simulink model "pilote_proportionnel_archive"  (R2018b)
settings: Solver=VariableStepAuto  StartTime=0.0  StopTime=10  MaxStep=0.01  RelTol=1e-3
undefined symbols (not defined in the file): alpha, beta, k, to
settings Model: Creator=12210406  LastModifiedBy=12210406

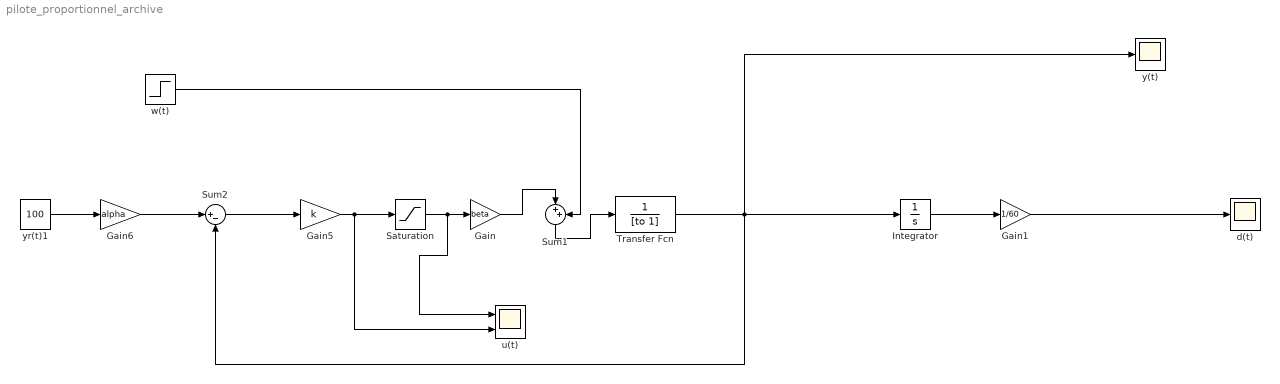
== system pilote_proportionnel_archive ==
  Gain : Gain  Gain=beta
  Gain1 : Gain  Gain=1/60
  Gain5 : Gain  Gain=k
  Gain6 : Gain  Gain=alpha
  Integrator : Integrator  LimitOutput=on  UpperSaturationLimit=t  LowerSaturationLimit=0
  Saturation : Saturate  UpperLimit=100  LowerLimit=-50
  Sum1 : Sum  Inputs=|++
  Sum2 : Sum  Inputs=|+-
  Transfer Fcn : TransferFcn  Denominator=[to 1]
  d(t) : Scope
  u(t) : Scope  NumInputPorts=2
  "w(t) " : Step  After=-10  SampleTime=0
  y(t) : Scope
  yr(t)1 : Constant  Value=100
  wires:
  Transfer Fcn/1 -> y(t)/1, Integrator/1, Sum2/2
  Integrator/1 -> Gain1/1
  Gain1/1 -> d(t)/1
  Saturation/1 -> u(t)/1, Gain/1
  Gain6/1 -> Sum2/1
  yr(t)1/1 -> Gain6/1
  Sum2/1 -> Gain5/1
  Gain5/1 -> u(t)/2, Saturation/1
  Gain/1 -> Sum1/1
  Sum1/1 -> Transfer Fcn/1
  "w(t) "/1 -> Sum1/2
